simulink subsystem "FixedWingScheduler"  (R2023b)
settings: Solver=VariableStepAuto  StartTime=0.0  StopTime=10.0  RelTol=1e-3
settings Model: Creator=The MathWorks, Inc.  LastModifiedBy=The MathWorks, Inc.

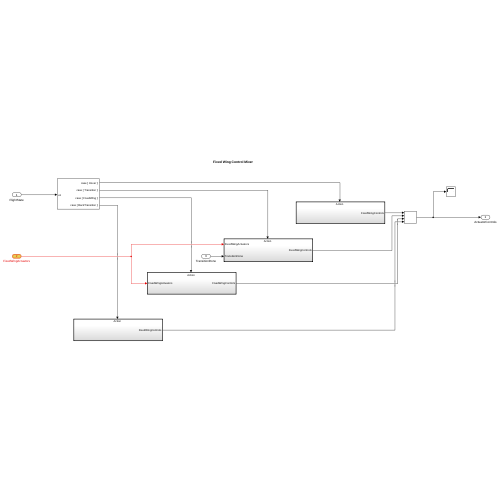
[thumbnail: Simulink's stored preview of the top-level diagram]
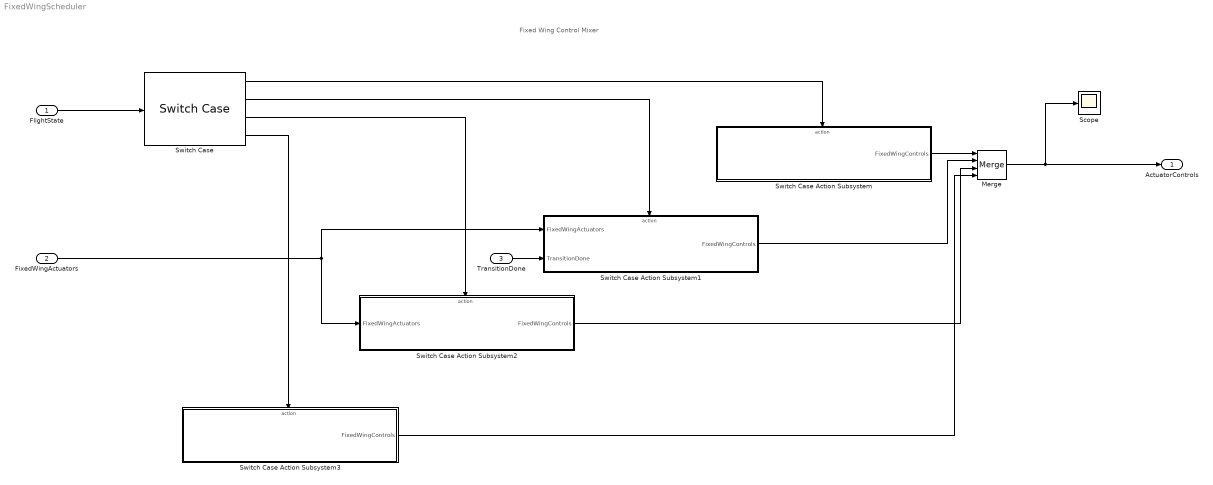
== system FixedWingScheduler ==
  note: Fixed Wing Control Mixer
  FlightState : Inport
  FixedWingActuators : Inport  Port=2  OutDataTypeStr=Bus: FixedWingCtrlBus
  TransitionDone : Inport  Port=3
  Merge : Merge  Inputs=4
  Scope : Scope
  Switch Case : SwitchCase  CaseConditions={flightState.Hover, flightState.Transition, flightState.FixedWing,flightState.BackTransition}  ShowDefaultCase=off
  Switch Case Action Subsystem : Subsystem  TreatAsAtomicUnit=on
  Switch Case Action Subsystem1 : Subsystem  TreatAsAtomicUnit=on
  Switch Case Action Subsystem2 : Subsystem  TreatAsAtomicUnit=on
  Switch Case Action Subsystem3 : Subsystem  TreatAsAtomicUnit=on
  ActuatorControls : Outport
  wires:
  FixedWingActuators/1 -> Switch Case Action Subsystem1/1(FixedWingActuators), Switch Case Action Subsystem2/1(FixedWingActuators)
  Merge/1 -> ActuatorControls/1, Scope/1
  Switch Case Action Subsystem2/1(FixedWingControls) -> Merge/3
  Switch Case Action Subsystem/1(FixedWingControls) -> Merge/1
  Switch Case/1 -> Switch Case Action Subsystem/Action
  Switch Case/2 -> Switch Case Action Subsystem1/Action
  Switch Case/3 -> Switch Case Action Subsystem2/Action
  Switch Case Action Subsystem1/1(FixedWingControls) -> Merge/2
  FlightState/1 -> Switch Case/1
  TransitionDone/1 -> Switch Case Action Subsystem1/2(TransitionDone)
  Switch Case/4 -> Switch Case Action Subsystem3/Action
  Switch Case Action Subsystem3/1(FixedWingControls) -> Merge/4

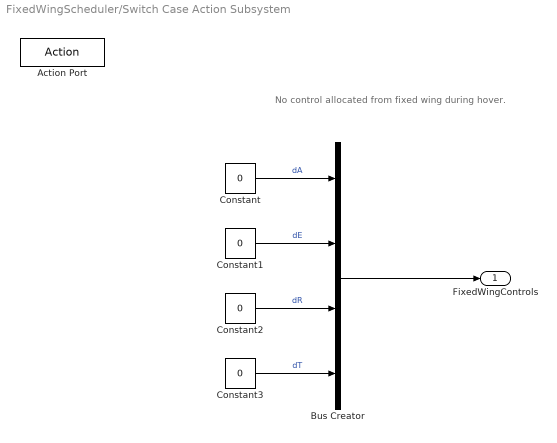
== system FixedWingScheduler/Switch Case Action Subsystem ==
  note: No control allocated from fixed wing during hover.
  Action Port : ActionPort
  Bus Creator : BusCreator  Inputs=4
  Constant{,1..3} (4 alike) : Constant  Value=0
  FixedWingControls : Outport  OutDataTypeStr=Bus: FixedWingCtrlBus
  wires:
  Constant3/1 -> Bus Creator/4  "dT"
  Constant2/1 -> Bus Creator/3  "dR"
  Constant1/1 -> Bus Creator/2  "dE"
  Constant/1 -> Bus Creator/1  "dA"
  Bus Creator/1 -> FixedWingControls/1

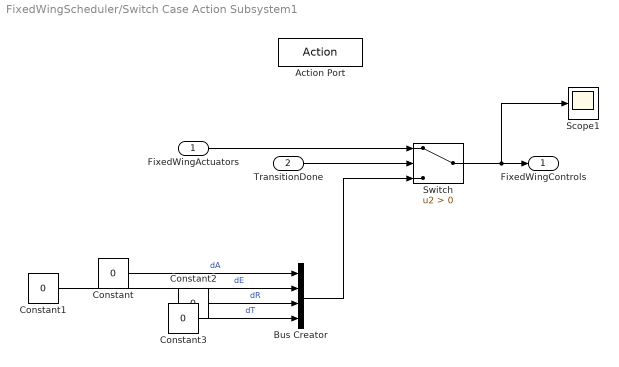
== system FixedWingScheduler/Switch Case Action Subsystem1 ==
  FixedWingActuators : Inport  OutDataTypeStr=Bus: FixedWingCtrlBus
  TransitionDone : Inport  Port=2
  Action Port : ActionPort
  Bus Creator : BusCreator  Inputs=4  OutDataTypeStr=Bus: FixedWingCtrlBus
  Constant{,1..3} (4 alike) : Constant  Value=0
  Scope1 : Scope
  Switch : Switch  Criteria=u2 > Threshold  SaturateOnIntegerOverflow=off  InputSameDT=off
  FixedWingControls : Outport  OutDataTypeStr=Bus: FixedWingCtrlBus
  wires:
  TransitionDone/1 -> Switch/2
  Switch/1 -> FixedWingControls/1, Scope1/1
  FixedWingActuators/1 -> Switch/1
  Constant3/1 -> Bus Creator/4  "dT"
  Constant2/1 -> Bus Creator/3  "dR"
  Constant1/1 -> Bus Creator/2  "dE"
  Constant/1 -> Bus Creator/1  "dA"
  Bus Creator/1 -> Switch/3

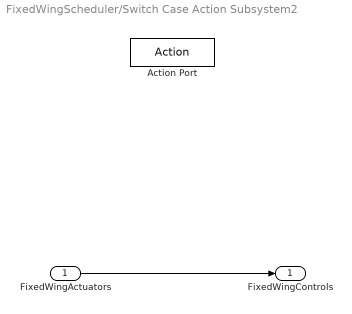
== system FixedWingScheduler/Switch Case Action Subsystem2 ==
  FixedWingActuators : Inport  OutDataTypeStr=Bus: FixedWingCtrlBus
  Action Port : ActionPort
  FixedWingControls : Outport  OutDataTypeStr=Bus: FixedWingCtrlBus
  wires:
  FixedWingActuators/1 -> FixedWingControls/1

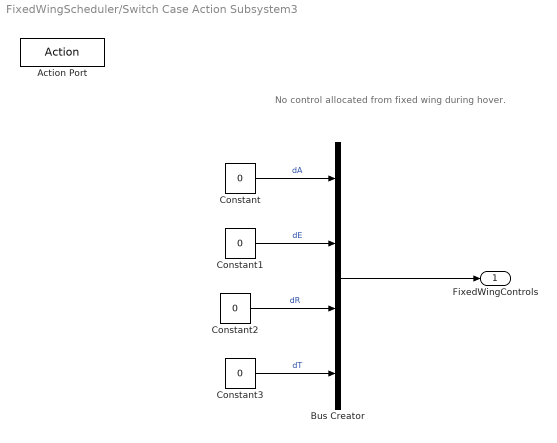
== system FixedWingScheduler/Switch Case Action Subsystem3 ==
  note: No control allocated from fixed wing during hover.
  Action Port : ActionPort
  Bus Creator : BusCreator  Inputs=4
  Constant{,1..3} (4 alike) : Constant  Value=0
  FixedWingControls : Outport  OutDataTypeStr=Bus: FixedWingCtrlBus
  wires:
  Constant2/1 -> Bus Creator/3  "dR"
  Constant3/1 -> Bus Creator/4  "dT"
  Constant1/1 -> Bus Creator/2  "dE"
  Constant/1 -> Bus Creator/1  "dA"
  Bus Creator/1 -> FixedWingControls/1
